simulink model "task8_lab13"  (R2021a)
settings: Solver=VariableStepAuto  StartTime=0.0  StopTime=10.0  RelTol=1e-3
settings Model: Creator=reemb  LastModifiedBy=reemb

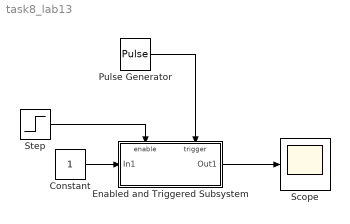
== system task8_lab13 ==
  Constant : Constant
  Enabled and Triggered Subsystem : Subsystem  TreatAsAtomicUnit=on
  Pulse Generator : DiscretePulseGenerator  PulseType=Time based  Period=1  PulseWidth=50
  Scope : Scope
  Step : Step  Time=3  SampleTime=0
  wires:
  Enabled and Triggered Subsystem/1(Out1) -> Scope/1
  Step/1 -> Enabled and Triggered Subsystem/Enable
  Pulse Generator/1 -> Enabled and Triggered Subsystem/Trigger
  Constant/1 -> Enabled and Triggered Subsystem/1(In1)

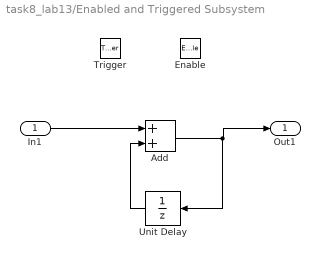
== system task8_lab13/Enabled and Triggered Subsystem ==
  In1 : Inport
  Enable : EnablePort
  Trigger : TriggerPort  VariantControl=(inherit)
  Add : Sum
  Unit Delay : UnitDelay  SampleTime=-1  HasFrameUpgradeWarning=on
  Out1 : Outport
  wires:
  In1/1 -> Add/1
  Unit Delay/1 -> Add/2
  Add/1 -> Unit Delay/1, Out1/1
